simulink model "CDSBasic"  (R2018b)
settings: Solver=FixedStepDiscrete  StartTime=0.0  StopTime=10.0  FixedStep=0.1  RelTol=1e-3
PreLoadFcn:
  | load test_data.mat;
settings Model: Creator=slentine  LastModifiedBy=wstuart
settings DataIOCC: SaveFormat=StructureWithTime
settings OptimizationCC: BlockReduction=off  DefaultParameterBehavior=Inlined  EnhancedBackFolding=on  PassReuseOutputArgsAs=Individual arguments  OptimizeBlockOrder=speed  DifferentSizesBufferReuse=on  OptimizationCustomize=off
settings DebuggingCC: ParameterTunabilityLossMsg=error
settings SFSimCC: MATLABDynamicMemAlloc=off
settings RTWCC: SystemTargetFile=cfs_ert.tlc  TemplateMakefile=ert_default_tmf  Description=NASA CFS Target File  GenerateReport=on  IncludeHyperlinkInReport=on  LaunchReport=on  PortableWordSizes=on  GenerateTraceInfo=on  GenerateTraceReport=on  GenerateTraceReportSl=on  GenerateTraceReportSf=on  GenerateTraceReportEml=on
settings CodeAppCC: ForceParamTrailComments=on  IgnoreCustomStorageClasses=off  OperatorAnnotations=on  SimulinkDataObjDesc=on  SFDataObjDesc=on  InsertBlockDesc=on
settings STFCustomTargetCC: TargetLangStandard=C99 (ISO)  MultiwordLength=256  GenerateSampleERTMain=on  CombineOutputUpdateFcns=on  ERTCustomFileBanners=on  SupportContinuousTime=off  SupportNonInlinedSFcns=off  RemoveResetFunc=on  SupportVariableSizeSignals=on  MATLABClassNameForMDSCustomization=Simulink.SoftwareTarget.ERTCustomization  UseToolchainInfoCompliant=on  SystemTargetFile=cfs_ert.tlc
settings ERTTargetCC: TargetLangStandard=C99 (ISO)  GenerateSampleERTMain=on  ParMdlRefBuildCompliant=off  CompOptLevelCompliant=off  ConcurrentExecutionCompliant=off  SupportVariableSizeSignals=on  ModelStepFunctionPrototypeControlCompliant=off  CPPClassGenCompliant=off  InlinedParameterPlacement=NonHierarchical  ERTCustomFileTemplate=cfs_interface.tlc

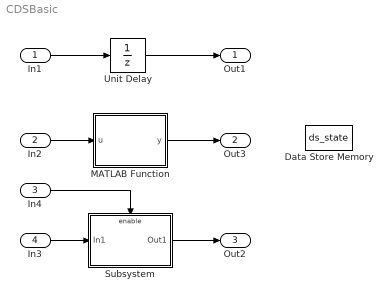
== system CDSBasic ==
  In1 : Inport  OutDataTypeStr=double  BusOutputAsStruct=on
  In2 : Inport  Port=2  OutDataTypeStr=int8  PortDimensions=35
  In4 : Inport  Port=3  Interpolate=off
  In3 : Inport  Port=4  OutDataTypeStr=single  PortDimensions=100  Interpolate=off
      settings: VarSizeSig=Yes
  Data Store Memory : DataStoreMemory  DataStoreName=ds_state  ReadBeforeWriteMsg=warning  WriteAfterWriteMsg=warning  WriteAfterReadMsg=warning  ShowAdditionalParam=off  OutDataTypeStr=int8  Dimensions=35
  MATLAB Function : MATLAB Function  TreatAsAtomicUnit=on
  Subsystem : Subsystem
  Unit Delay : UnitDelay  SampleTime=-1  StateName=state1  StateMustResolveToSignalObject=on
  Out1 : Outport  OutDataTypeStr=double  BusOutputAsStruct=on
  Out3 : Outport  Port=2  OutDataTypeStr=int8  BusOutputAsStruct=on
  Out2 : Outport  Port=3  BusOutputAsStruct=on
  wires:
  In1/1 -> Unit Delay/1
  MATLAB Function/1(y) -> Out3/1
  Unit Delay/1 -> Out1/1
  In2/1 -> MATLAB Function/1(u)
  In3/1 -> Subsystem/1(In1)
  Subsystem/1(Out1) -> Out2/1
  In4/1 -> Subsystem/Enable

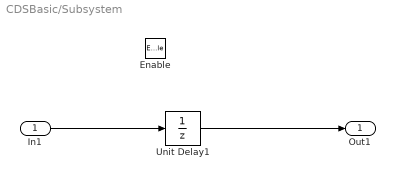
== system CDSBasic/Subsystem ==
  In1 : Inport
  Enable : EnablePort  StatesWhenEnabling=reset
  Unit Delay1 : UnitDelay  SampleTime=-1  StateName=state2
  Out1 : Outport
  wires:
  Unit Delay1/1 -> Out1/1
  In1/1 -> Unit Delay1/1

== matlab function CDSBasic/MATLAB Function ==
  data: u input; y output; ds_state data_store_memory
function y = fcn(u) %#codegen
persistent ds_state;

if isempty(ds_state)
    ds_state = zeros(35,1,'int8');
end
y = ds_state;
ds_state  = u;
